simulink model "Full_Wave_Rectifier_HalfControlled_Rload2015"  (R2015a)
settings: Solver=ode45  SolverMode=SingleTasking  StartTime=0.0  StopTime=0.06  RelTol=1e-3
undefined symbols (not defined in the file): powergui
libraries: powerlib x13
settings Model: CovMetricSettings=dwe  CovHtmlReporting=off  covSaveCumulativeToWorkspaceVar=off  CovSaveSingleToWorkspaceVar=off  CovExternalEMLEnable=on  Creator=A.hey  LastModifiedBy=A.hey
settings DataIOCC: LimitDataPoints=off  SaveFormat=Dataset
settings DebuggingCC: SFUnexpectedBacktrackingDiag=error  SFNoUnconditionalDefaultTransitionDiag=error
settings HardwareCC: ProdBitPerPointer=64  ProdLargestAtomicFloat=Float  ProdIntDivRoundTo=Zero  ProdEndianess=LittleEndian  ProdHWDeviceType=Specified
settings ModelReferenceCC: PropagateSignalLabelsOutOfModel=on
settings SFSimCC: SimUseLocalCustomCode=on
settings RTWCC: RTWUseLocalCustomCode=on
settings GRTTargetCC: TargetLangStandard=C99 (ISO)  GeneratePreprocessorConditionals=Use local settings
settings ConfigurationSet: Description=Simscape Multibody

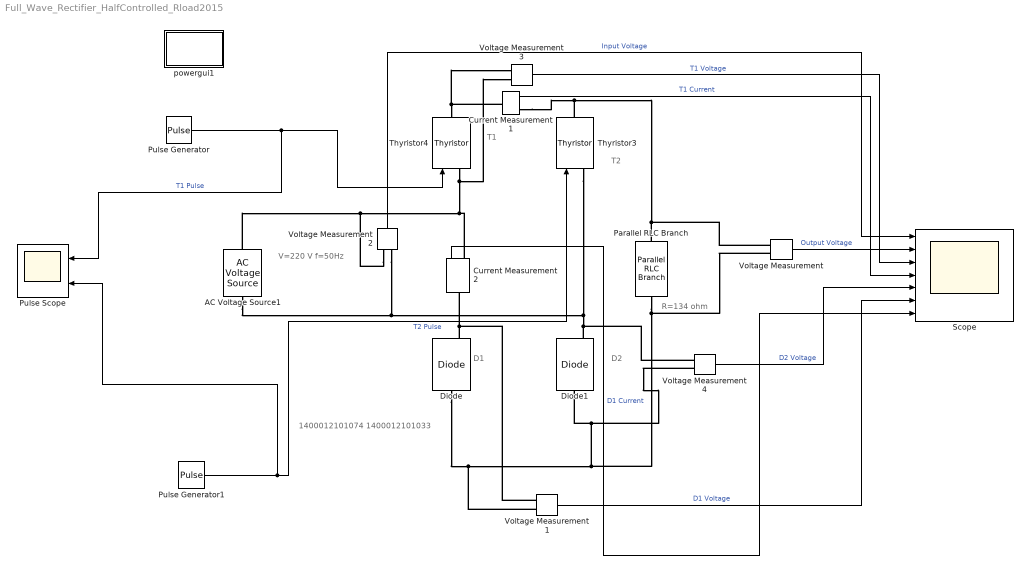
== system Full_Wave_Rectifier_HalfControlled_Rload2015 ==
  note: D2
  note: T1
  note: V=220 V
      | f=50Hz
  note: D1
  note: T2
  note: R=134 ohm
  note: 1400012101074
      | 1400012101033
  AC Voltage Source1 : powerlib/Electrical Sources/AC Voltage Source  Amplitude=220  Phase=0  Frequency=50  SampleTime=0  Measurements=None  BusType=swing  Pref=10e3  Qref=0  Qmin=-inf  Qmax=+inf
  Current Measurement1 : powerlib/Measurements/Current Measurement  PhasorSimulation=off  OutputType=Complex  PSBequivalent=0
  Current Measurement2 : powerlib/Measurements/Current Measurement  PhasorSimulation=off  OutputType=Complex  PSBequivalent=0
  Diode : powerlib/Power Electronics/Diode  Ron=0.001  Lon=0  Vf=0.8  IC=0  UseSnubber=0  Rs=500  Cs=250e-9  Measurements=on
  Diode1 : powerlib/Power Electronics/Diode  Ron=0.001  Lon=0  Vf=0.8  IC=0  UseSnubber=0  Rs=500  Cs=250e-9  Measurements=on
  Parallel RLC Branch : powerlib/Elements/Parallel RLC Branch  LConnTagsString=a  RConnTagsString=__new0  BranchType=R  Resistance=134  Inductance=1e-3  SetiL0=off  InitialCurrent=0  Capacitance=1e-6  Setx0=off  InitialVoltage=0  Measurements=None
  Pulse Generator : DiscretePulseGenerator  PulseType=Time based  Amplitude=10  Period=0.02  PulseWidth=25  PhaseDelay=0.005
  Pulse Generator1 : DiscretePulseGenerator  PulseType=Time based  Amplitude=10  Period=0.02  PulseWidth=25  PhaseDelay=0.015
  Pulse Scope : Scope  NumInputPorts=2
      settings: TimeRange=auto  ShowLegends=on  MaxDataPoints=5000  SaveToWorkspace=off  YMin=-1.25~-1.25  YMax=11.25~11.25  SampleTime=-1
  "Scope " : Scope  NumInputPorts=7
      settings: TimeRange=auto  ShowLegends=on  MaxDataPoints=5000  SaveToWorkspace=off  SaveName=ScopeData  YMin=-275.00000~-27.38698~-274.76726~-0.75155~-246.7002~-246.7002~-0.22358  YMax=275.00000~246.48284~273.93041~2.38659~28.30184~28.30184~1.84233  SampleTime=-1
  Thyristor3 : powerlib/Power Electronics/Thyristor  Ron=0.001  Lon=0  Vf=0.1  IC=0  Rs=500  Cs=250e-9  Measurements=off
  Thyristor4 : powerlib/Power Electronics/Thyristor  Ron=0.001  Lon=0  Vf=0.1  IC=0  Rs=500  Cs=250e-9  Measurements=off
  Voltage Measurement{,1..4} (5 alike) : powerlib/Measurements/Voltage Measurement  PhasorSimulation=off  OutputType=Complex  PSBequivalent=0
  powergui1 : Subsystem  Priority=1  AncestorBlock=powerlib/powergui  DialogController=POWERSYS.PowerSysDialog  InitFcn=powergui( 'InitFcn_Callback' , gcb , 0 , [ ] );  mask(PSB option menu block){SimulationMode=Continuous, SampleTime=50e-6, frequency=60, Iterations=50, frequencyindice=50, Pbase=100e6, ErrMax=1e-4, UnitsV=kV, UnitsW=MW, buscounter=0, FunctionMessages=off, echomessages=off, EnableUseOfTLC=off, CurrentSourceSwitches=off, DisableSnubberDevices=off, DisableRonSwitches=off, DisableVfSwitches=off, DisplayEquations=off, SolverType=Tustin/Backward Euler (TBE), Interpol=off, ExternalGateDelay=off, methode=off, Ts=100, x0status=blocks, SPID=on, SwTol=0, HookPort=off, RestoreLinks=warning, ResistiveCurrentMeasurement=off, Frange=[0:2:500], Ylog=off, Xlog=on, ShowGrid=off, save=off, variable=ZData, structure=0, ZoomFFT=off, StartTime=0.0, cycles=1, DisplayStyle=1, fundamental=60, FreqAxis=off, MaxFrequency=1000, frequencyindicesteady=1, RmsSteady=1, display=off}
      mask prompts: SimulationMode "Simulation type:"; SampleTime "Sample time (s):"; frequency "Frequency (Hz):"; Iterations "Max iterations"; frequencyindice "Frequency (Hz)"; Pbase "Base power (VA)"; ErrMax "PQ tolerance (pu)"; UnitsV "Voltage units"; UnitsW "Power units"; buscounter "Load flow bus counter"; FunctionMessages "Disable Specialized Power Systems warnings"; echomessages "Display Specialized Power Systems compilation messages"; EnableUseOfTLC "Use TLC file when in Accelerator Simulation Mode and for code generation"; CurrentSourceSwitches "Disable ideal switching"; DisableSnubberDevices "Disable snubbers in switching devices"; DisableRonSwitches "Disable Ron resistances in switching devices"; DisableVfSwitches "Disable forward voltages in switching devices"; DisplayEquations "Display circuit differential equations"; SolverType "Discrete solver"; Interpol "Interpolate switching events"; ExternalGateDelay "Use time-stamped gate signals"; methode "Store switching topologies"; Ts "Buffer size (MBytes):"; x0status "Start simulation with initial electrical states from:"; SPID "Use ideal switching devices"; SwTol "Switch tolerance"; HookPort "Allow multiple powergui blocks"; RestoreLinks "Restore disabled links of Simscape Power Systems ST blocks:"; ResistiveCurrentMeasurement "Use non ideal current measurement blocks (1e-4Ohm internal resistance)"; Frange "Frequency Range"; Ylog "Log impedance"; Xlog "log Frequency"; ShowGrid "grid"; save "Save Data To Workspace"; variable "Variable Name"; structure "Structure Name (PSBFFTSCOPE)"; ZoomFFT "ZoomFFT (PSBFFTSCOPE)"; StartTime "Start Time (PSBFFTSCOPE)"; cycles "Cycles (PSBFFTSCOPE)"; DisplayStyle "Display style (PSBFFTSCOPE)"; fundamental "Fundamental (PSBFFTSCOPE)"; FreqAxis "Frequency Axis (PSBFFTSCOPE)"; MaxFrequency "Max Frequency (PSBFFTSCOPE)"; frequencyindicesteady "Frequency indice (STEADYSTATE)"; RmsSteady "RMS display (STEADYSTATE)"; display "Display Results"
      mask help: Set simulation type, simulation parameters, and preferences.
      mask init:
      | dispMessage = powergui('MaskInitialization',gcb,SimulationMode,SampleTime);
      settings: PreSaveFcn=powergui( 'PreSaveFcn_Callback' , gcb , [ ] , [ ] );  OpenFcn=sps_rtmsupport('OpenFcn',gcbh)
      mask Help: helpview(psbhelp)
      mask TypeOptions SimulationMode: Continuous | Discrete | Phasor
      mask Callback SimulationMode: powergui('SimulationType',[],[],gcb);
      mask TypeOptions UnitsV: V | kV
      mask TypeOptions UnitsW: W | kW | MW
      mask Callback CurrentSourceSwitches: powergui('SimulationType',[],[],gcb);
      mask TypeOptions SolverType: Tustin/Backward Euler (TBE) | Tustin | Backward Euler
      mask Callback SolverType: powergui('SimulationType',[],[],gcb);
      mask Callback Interpol: powergui('SimulationType',[],[],gcb);
      mask Callback ExternalGateDelay: powergui('SimulationType',[],[],gcb);
      mask Callback methode: powergui('SimulationType',[],[],gcb);
      mask TypeOptions x0status: blocks | steady | zero
      mask TypeOptions RestoreLinks: yes | warning | no
      mask Callback display: sps_rtmsupport('parametereditingmodes',gcbh) % Will be executed last in parameter callbacks to ensure mask enable consistency
      mask DialogControl AutoSolverNote Prompt: To enable the Powergui solver settings, unselect auto (Automatic solver selection) solver in the Simulink solver options.
      mask DialogControl SteadyState Prompt: Steady-State
      mask DialogControl SteadyState Callback: close_system(gcb); power_steadystate(bdroot(gcb),gcb);
      mask DialogControl InitialState Prompt: Initial State
      mask DialogControl InitialState Callback: close_system(gcb); power_initstates(bdroot(gcb),gcb)
      mask DialogControl MachineInitialization Prompt: Machine Initialization
      mask DialogControl MachineInitialization Callback: close_system(gcb); power_loadflow(bdroot(gcb),gcb);
      mask DialogControl ImpedanceMeasurement Prompt: Impedance Measurement
      mask DialogControl ImpedanceMeasurement Callback: close_system(gcb); power_zmeter(bdroot(gcb),gcb);
      mask DialogControl FFTAnalysis Prompt: FFT Analysis
      mask DialogControl FFTAnalysis Callback: close_system(gcb); power_fftscope(bdroot(gcb),gcb);
      mask DialogControl LinearSystemAnalyzer Prompt: Use Linear System Analyzer
      mask DialogControl LinearSystemAnalyzer Callback: close_system(gcb); power_ltiview(bdroot(gcb),gcb);
      mask DialogControl HysteresisDesign Prompt: Hysteresis Design
      mask DialogControl HysteresisDesign Callback: close_system(gcb); power_hysteresis(bdroot(gcb),gcb);
      mask DialogControl RLCLineParameters Prompt: RLC Line Parameters
      mask DialogControl RLCLineParameters Callback: close_system(gcb); power_lineparam(bdroot(gcb),gcb);
      mask DialogControl GenerateReprot Prompt: Generate Report
      mask DialogControl GenerateReprot Callback: close_system(gcb); power_report(bdroot(gcb),gcb);
      mask DialogControl Control14 Prompt: Customize SPS blocks
      mask DialogControl Control14 Callback: close_system(gcb); power_customize;
      mask DialogControl LoadFlow Prompt: Load Flow
      mask DialogControl LoadFlow Callback: close_system(gcb); power_loadflow('-v2',bdroot(gcb));
      mask DialogControl Container14 Prompt: Load flow settings
      mask Display: color('blue'),disp(dispMessage)
  wires:
  Voltage Measurement4/1 -> "Scope "/5  "D2 Voltage"
  Voltage Measurement1/1 -> "Scope "/6  "D1 Voltage"
  Pulse Generator/1 -> Pulse Scope/1, Thyristor4/1  "T1 Pulse"
  Voltage Measurement/1 -> "Scope "/2  "Output Voltage"
  Voltage Measurement3/1 -> "Scope "/3  "T1 Voltage"
  Current Measurement1/1 -> "Scope "/4  "T1 Current"
  Pulse Generator1/1 -> Thyristor3/1, Pulse Scope/2  "T2 Pulse"
  Voltage Measurement2/1 -> "Scope "/1  "Input Voltage"
  Current Measurement2/1 -> "Scope "/7  "D1 Current"
  connections:
  Voltage Measurement4/LConn2 -- Diode1/RConn1 -- Thyristor3/LConn1 -- Voltage Measurement2/LConn2 -- AC Voltage Source1/LConn1
  Current Measurement1/LConn1 -- Thyristor4/RConn1 -- Voltage Measurement3/LConn2
  Voltage Measurement4/LConn1 -- Diode1/LConn1 -- Diode/LConn1 -- Voltage Measurement1/LConn1 -- Parallel RLC Branch/RConn1 -- Voltage Measurement/LConn2
  Voltage Measurement1/LConn2 -- Current Measurement2/LConn1 -- Diode/RConn1
  Voltage Measurement/LConn1 -- Thyristor3/RConn1 -- Current Measurement1/RConn1 -- Parallel RLC Branch/LConn1
  AC Voltage Source1/RConn1 -- Voltage Measurement2/LConn1 -- Current Measurement2/RConn1 -- Thyristor4/LConn1 -- Voltage Measurement3/LConn1

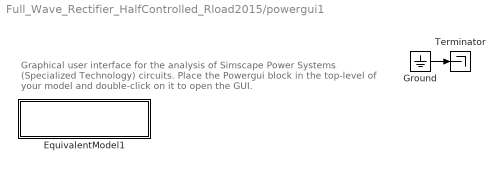
== system Full_Wave_Rectifier_HalfControlled_Rload2015/powergui1 ==
  note: Graphical user interface for the analysis of
      | Simscape Power Systems (Specialized Technology) circuits.
      | Place the Powergui block in the top-level of your model and double-click
      | on it to open the GUI.
  EquivalentModel1 : Subsystem  mask{SwTol=SwTol}
      mask prompts: SwTol "SwitchTolerance"
      mask init:
      | S  = GetDataForEquivalentModel('SPID',gcbh,SwTol);
      mask Display:
      | color('blue')
      | disp('EQUIVALENT CIRCUIT\nSPID')
  Ground : Ground
  Terminator : Terminator
  wires:
  Ground/1 -> Terminator/1

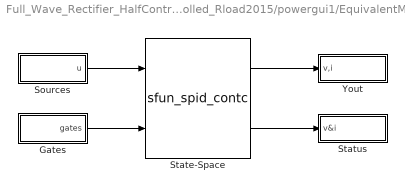
== system Full_Wave_Rectifier_HalfControlled_Rload2015/powergui1/EquivalentModel1 ==
  Gates : Subsystem
  Sources : Subsystem
  State-Space : S-Function  FunctionName=sfun_spid_contc  Parameters=S.Mg, [S.nb.x S.nb.u S.nb.y S.nb.s], S.x0, S.MgColNames, S.SwitchVf, S.SwitchType, S.SwitchGateInitialValue, S.SwitchTolerance,S.SaveMatrices,S.BufferSize  SFunctionDeploymentMode=off  EnableBusSupport=off
  Status : Subsystem
  Yout : Subsystem
  wires:
  State-Space/1 -> Yout/1(v,i)
  State-Space/2 -> Status/1(v&i)
  Gates/1(gates) -> State-Space/2
  Sources/1(u) -> State-Space/1

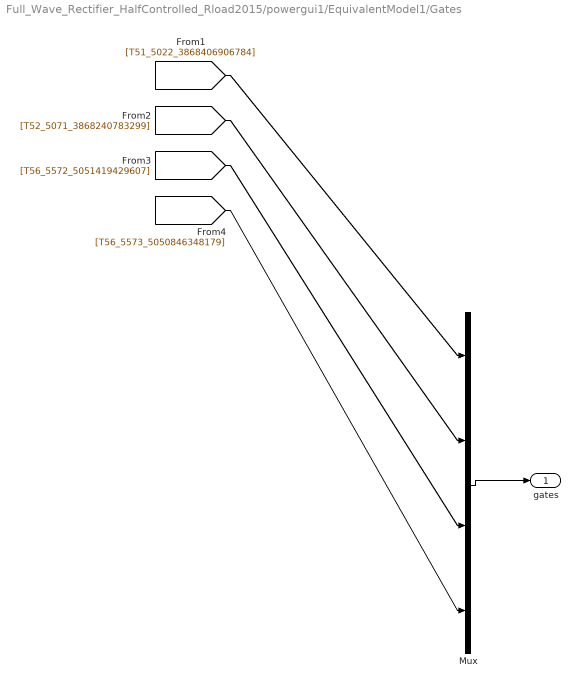
== system Full_Wave_Rectifier_HalfControlled_Rload2015/powergui1/EquivalentModel1/Gates ==
  Mux : Mux  Inputs=[1 1 1 1]
  gates : Outport
  wires:
  Mux/1 -> gates/1
  [T51_5022_3868406906784] -> Mux/1
  [T52_5071_3868240783299] -> Mux/2
  [T56_5572_5051419429607] -> Mux/3
  [T56_5573_5050846348179] -> Mux/4

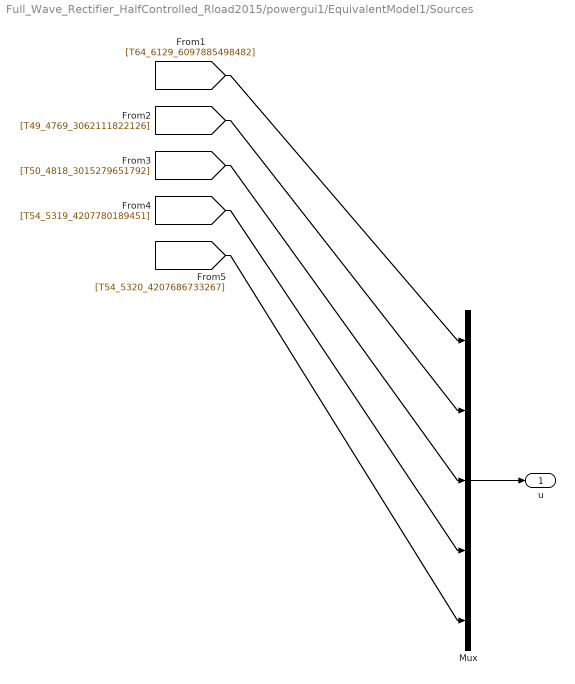
== system Full_Wave_Rectifier_HalfControlled_Rload2015/powergui1/EquivalentModel1/Sources ==
  Mux : Mux  Inputs=[1 1 1 1 1]
  u : Outport
  wires:
  Mux/1 -> u/1
  [T64_6129_6097885498482] -> Mux/1
  [T49_4769_3062111822126] -> Mux/2
  [T50_4818_3015279651792] -> Mux/3
  [T54_5319_4207780189451] -> Mux/4
  [T54_5320_4207686733267] -> Mux/5

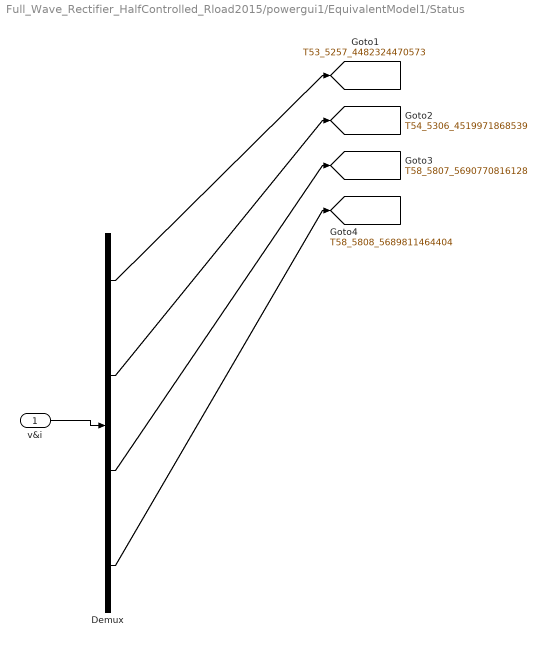
== system Full_Wave_Rectifier_HalfControlled_Rload2015/powergui1/EquivalentModel1/Status ==
  v&i : Inport
  Demux : Demux  Outputs=[2 2 2 2]
  tag scope: T53_5257_4482324470573=global, T54_5306_4519971868539=global, T58_5807_5690770816128=global, T58_5808_5689811464404=global
  wires:
  v&i/1 -> Demux/1
  Demux/1 -> [T53_5257_4482324470573]
  Demux/2 -> [T54_5306_4519971868539]
  Demux/3 -> [T58_5807_5690770816128]
  Demux/4 -> [T58_5808_5689811464404]

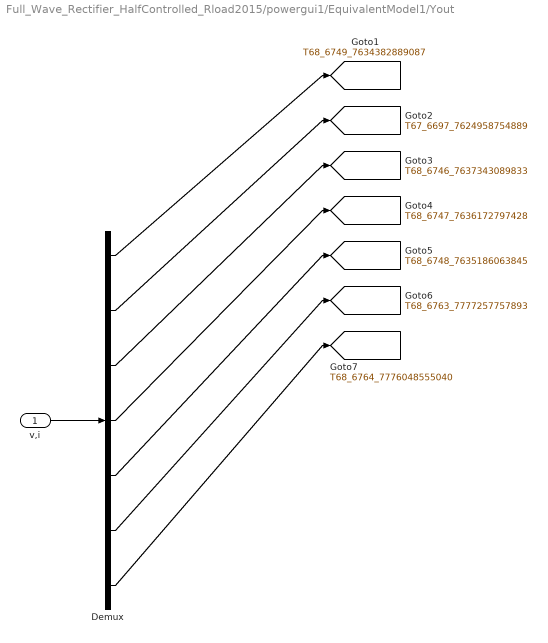
== system Full_Wave_Rectifier_HalfControlled_Rload2015/powergui1/EquivalentModel1/Yout ==
  v,i : Inport
  Demux : Demux  Outputs=[1 1 1 1 1 1 1]
  tag scope: T67_6697_7624958754889=global, T68_6746_7637343089833=global, T68_6747_7636172797428=global, T68_6748_7635186063845=global, T68_6749_7634382889087=global, T68_6763_7777257757893=global, T68_6764_7776048555040=global
  wires:
  v,i/1 -> Demux/1
  Demux/1 -> [T68_6749_7634382889087]
  Demux/2 -> [T67_6697_7624958754889]
  Demux/3 -> [T68_6746_7637343089833]
  Demux/4 -> [T68_6747_7636172797428]
  Demux/5 -> [T68_6748_7635186063845]
  Demux/6 -> [T68_6763_7777257757893]
  Demux/7 -> [T68_6764_7776048555040]
